simulink model "samplingcircuit"  (R2014a)
settings: Solver=ode3  StartTime=0.0  StopTime=20  FixedStep=1/(44100*16)  RelTol=1e-3
values from neighbouring files (symbols this model uses):
  quantBreak = lutix(2^bits)    [oversampling.m]
  quantData = lutdata(2^bits)    [oversampling.m]
libraries: simulink x1, dspsrcs4 x1, dspsigattribs x1, dsparch4 x1
settings Model: Creator=Administratör  LastModifiedBy=Administratör

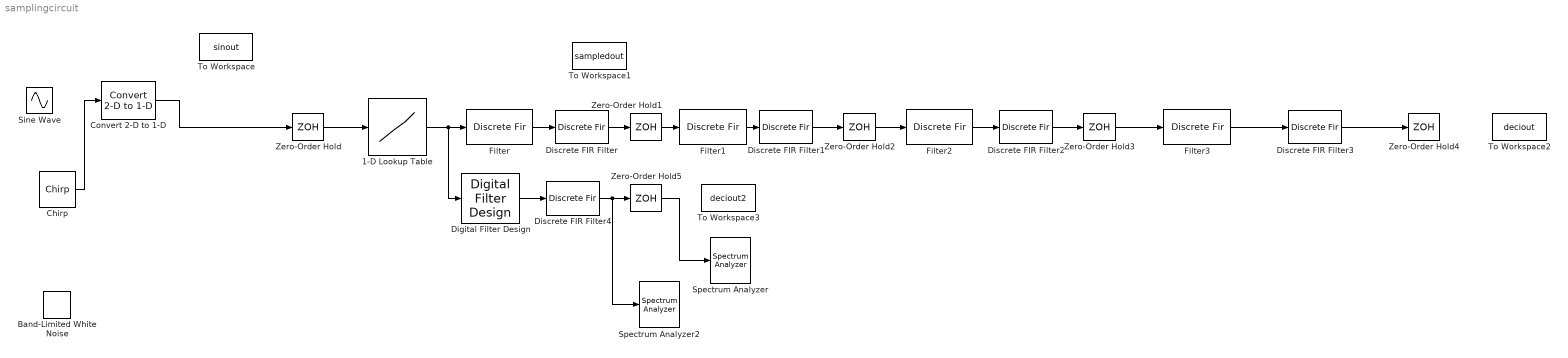
== system samplingcircuit ==
  1-D Lookup Table : Lookup_n-D  NumberOfTableDimensions=1  BreakpointsForDimension1=quantBreak  Table=quantData  InterpMethod=Flat  InternalRulePriority=Speed  RndMeth=Simplest  InputSameDT=on
  Band-Limited White Noise : simulink/Sources/Band-Limited White Noise  Cov=1  Ts=1/(44100*16)  seed=[23341]
  Chirp : dspsrcs4/Chirp  sweep=Logarithmic  mode=Unidirectional  f0=1000  f1=44100*8  t1=20  Tsweep=20  phase=0  Ts=1/(44100*16)  spf=1  datatype=Double
  Convert 2-D to 1-D : dspsigattribs/Convert 2-D to 1-D
  Digital Filter Design : dsparch4/Digital Filter Design  mwdsp_browser_bugfix_var=off
  Discrete FIR Filter{,1..3} (4 alike) : DiscreteFir
  Discrete FIR Filter4 : DiscreteFir  Coefficients=[1/16 1/16 1/16 1/16 1/16 1/16 1/16 1/16 1/16 1/16 1/16 1/16 1/16 1/16 1/16 1/16]
  Filter{,1..3} (4 alike) : DiscreteFir  Tag=BlockMethodSubSystem  Coefficients=[0.027363050980413479 0 -0.078643524359898201 0 0.30827197967917297 0.5 0.30827197967917297 0 -0.078643524359898201 0 0.027363050980413479]  InputProcessing=Columns as channels (frame based)
  Sine Wave : Sin  SampleTime=0
  Spectrum Analyzer : SpectrumAnalyzer
  Spectrum Analyzer2 : SpectrumAnalyzer
  To Workspace : ToWorkspace  VariableName=sinout  SaveFormat=Structure With Time  SampleTime=-1
  To Workspace1 : ToWorkspace  VariableName=sampledout  SaveFormat=Structure With Time  SampleTime=-1
  To Workspace2 : ToWorkspace  VariableName=deciout  SaveFormat=Structure With Time  SampleTime=-1
  To Workspace3 : ToWorkspace  VariableName=deciout2  SaveFormat=Structure With Time  SampleTime=-1
  Zero-Order Hold : ZeroOrderHold  SampleTime=1/(44100*16)
  Zero-Order Hold1 : ZeroOrderHold  SampleTime=1/(44100*8)
  Zero-Order Hold2 : ZeroOrderHold  SampleTime=1/(44100*4)
  Zero-Order Hold3 : ZeroOrderHold  SampleTime=1/(44100*2)
  Zero-Order Hold4 : ZeroOrderHold  SampleTime=1/(44100)
  Zero-Order Hold5 : ZeroOrderHold  SampleTime=1/(44100)
  wires:
  Zero-Order Hold/1 -> 1-D Lookup Table/1
  Discrete FIR Filter/1 -> Zero-Order Hold1/1
  Discrete FIR Filter1/1 -> Zero-Order Hold2/1
  Discrete FIR Filter2/1 -> Zero-Order Hold3/1
  Zero-Order Hold3/1 -> Filter3/1
  Discrete FIR Filter3/1 -> Zero-Order Hold4/1
  Convert 2-D to 1-D/1 -> Zero-Order Hold/1
  Discrete FIR Filter4/1 -> Zero-Order Hold5/1, Spectrum Analyzer2/1
  Zero-Order Hold5/1 -> Spectrum Analyzer/1
  Chirp/1 -> Convert 2-D to 1-D/1
  1-D Lookup Table/1 -> Filter/1, Digital Filter Design/1
  Digital Filter Design/1 -> Discrete FIR Filter4/1
  Filter/1 -> Discrete FIR Filter/1
  Zero-Order Hold1/1 -> Filter1/1
  Filter1/1 -> Discrete FIR Filter1/1
  Zero-Order Hold2/1 -> Filter2/1
  Filter2/1 -> Discrete FIR Filter2/1
  Filter3/1 -> Discrete FIR Filter3/1
